simulink model "dsss"  (Simulink 5.0)
settings: Solver=ode45  StartTime=0.0  StopTime=40.0  RelTol=1e-3
libraries: dspsigops x4, dsparch4 x2, commseqgen2 x2, commrandsrc2 x1
settings Model: LastModifiedBy=Daiming Qu

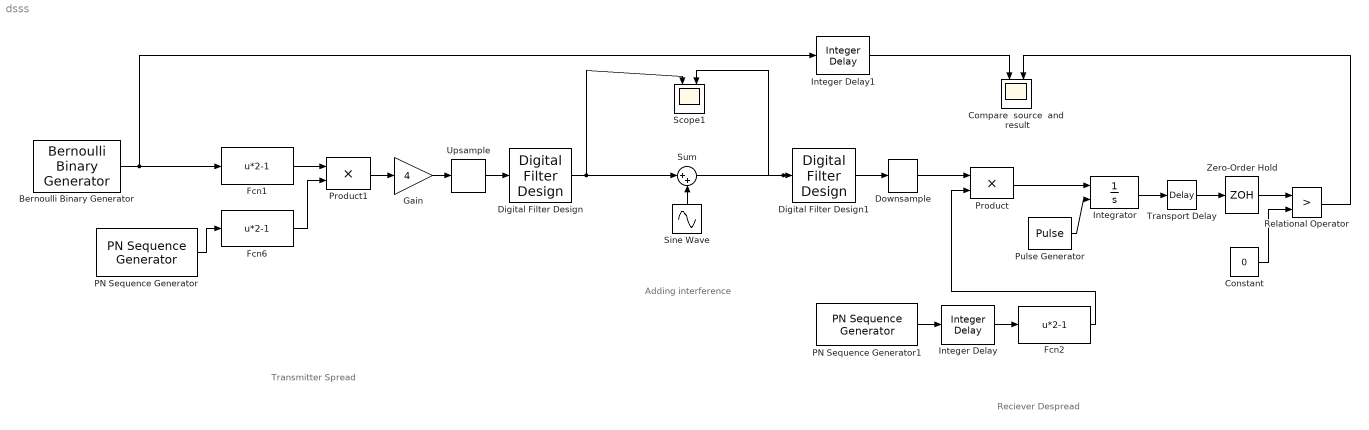
== system dsss ==
  note: Reciever
      | Despread
  note: Transmitter
      | Spread
  note: Adding interference
  Bernoulli Binary Generator : commrandsrc2/Bernoulli Binary Generator  P=0.5  seed=61  Ts=1  frameBased=off  sampPerFrame=1  orient=off
  Compare  source  and  result : Scope  NumInputPorts=2
      settings: Orientation=down  TimeRange=1.12079701120797  YMin=-0.5~-0.5  YMax=1.5~1.5
  Constant : Constant  Value=0
  Digital Filter Design : dsparch4/Digital Filter Design
  Digital Filter Design1 : dsparch4/Digital Filter Design
  Downsample : dspsigops/Downsample  N=4  phase=0  ic=0  smode=Allow multirate  fmode=Maintain input frame size
  Fcn1 : Fcn  Expr=u*2-1
  Fcn2 : Fcn  Expr=u*2-1
  Fcn6 : Fcn  Expr=u*2-1
  Gain : Gain  Gain=4  SaturateOnIntegerOverflow=on
  Integer Delay : dspsigops/Integer Delay  delay=12  ic=0  reset_popup=None
  Integer Delay1 : dspsigops/Integer Delay  delay=2  ic=0  reset_popup=None
  Integrator : Integrator  ExternalReset=rising
  PN Sequence Generator : commseqgen2/PN Sequence Generator  poly=[1 0 0 0 0 1 1]  ini_sta=[0 0 0 0 0 1]  shift=0  Ts=0.01  frameBased=off  sampPerFrame=1  reset=off
  PN Sequence Generator1 : commseqgen2/PN Sequence Generator  poly=[1 0 0 0 0 1 1]  ini_sta=[0 0 0 0 0 1]  shift=0  Ts=0.01  frameBased=off  sampPerFrame=1  reset=off
  Product : Product  SaturateOnIntegerOverflow=on
  Product1 : Product  SaturateOnIntegerOverflow=on
  Pulse Generator : DiscretePulseGenerator  PulseType=Time based  Period=1  PulseWidth=50  PhaseDelay=0.12
  Relational Operator : RelationalOperator  Operator=>
  Scope1 : Scope  NumInputPorts=2
      settings: Orientation=down  TimeRange=1.12079701120797  YMin=-2~-2  YMax=2~2
  Sine Wave : Sin  Orientation=up  Amplitude=4  SampleTime=1/400
  Sum : Sum  Inputs=|++  SaturateOnIntegerOverflow=on
  Transport Delay : TransportDelay  DelayTime=0.89
  Upsample : dspsigops/Upsample  N=4  phase=0  ic=0  mode=Maintain input frame size
  Zero-Order Hold : ZeroOrderHold
  wires:
  Upsample/1 -> Digital Filter Design/1
  Downsample/1 -> Product/1
  PN Sequence Generator1/1 -> Integer Delay/1
  Digital Filter Design/1 -> Sum/1, Scope1/1
  Digital Filter Design1/1 -> Downsample/1
  Sum/1 -> Scope1/2, Digital Filter Design1/1
  Bernoulli Binary Generator/1 -> Fcn1/1, Integer Delay1/1
  PN Sequence Generator/1 -> Fcn6/1
  Product/1 -> Integrator/1
  Zero-Order Hold/1 -> Relational Operator/1
  Pulse Generator/1 -> Integrator/2
  Relational Operator/1 -> Compare  source  and  result/2
  Fcn6/1 -> Product1/2
  Fcn1/1 -> Product1/1
  Sine Wave/1 -> Sum/2
  Integer Delay/1 -> Fcn2/1
  Fcn2/1 -> Product/2
  Constant/1 -> Relational Operator/2
  Integrator/1 -> Transport Delay/1
  Transport Delay/1 -> Zero-Order Hold/1
  Integer Delay1/1 -> Compare  source  and  result/1
  Product1/1 -> Gain/1
  Gain/1 -> Upsample/1
